simulink model "ssc_1C_Model_NT_MATLABfunc_est"  (R2019a)
settings: Solver=VariableStepAuto  StartTime=0  StopTime=150  FixedStep=0.05  RelTol=1e-4
undefined symbols (not defined in the file): C1_LUT, Capacity, Em_LUT, h, R0_LUT, R1_LUT, sigbuilder_block, SOC_LUT
libraries: nesl_utility x8, fl_lib x3
settings Model: OrderedModelArguments=off  Creator=ekonu001  LastModifiedBy=ekonu001
settings DataIOCC: ExternalInput=t

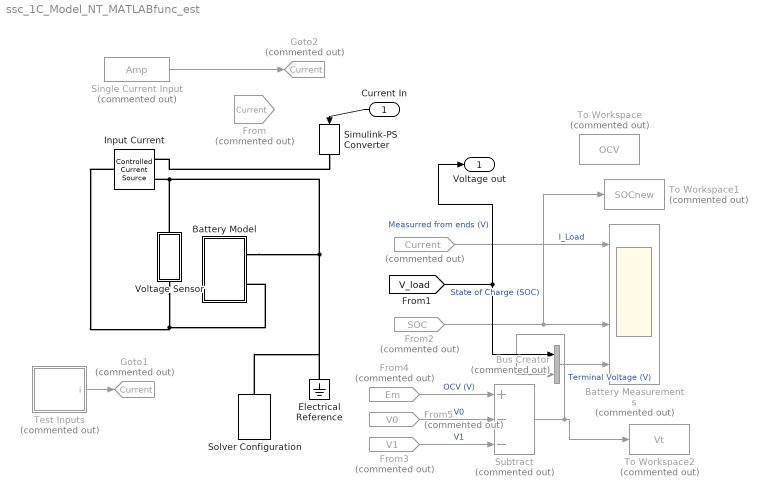
== system ssc_1C_Model_NT_MATLABfunc_est ==
  Current In : Inport
  " " : From  Commented=on  GotoTag=Current  TagVisibility=global
  Battery Measurements : Scope  Commented=on  NumInputPorts=4
  "Battery Model " : Subsystem
  Bus Creator : BusCreator  Commented=on  Inputs=2
  Electrical Reference : fl_lib/Electrical/Electrical Elements/Electrical Reference
  From : From  Commented=on  GotoTag=Current  TagVisibility=global
  From2 : From  Commented=on  GotoTag=SOC  TagVisibility=global
  From3 : From  Commented=on  GotoTag=V1  TagVisibility=global
  From4 : From  Commented=on  GotoTag=Em  TagVisibility=global
  From5 : From  Commented=on  GotoTag=V0  TagVisibility=global
  Goto1 : Goto  Commented=on  GotoTag=Current  TagVisibility=global
  Goto2 : Goto  Commented=on  GotoTag=Current  TagVisibility=global
  Input Current : fl_lib/Electrical/Electrical Sources/Controlled Current Source
  Simulink-PS Converter : nesl_utility/Simulink-PS Converter  PhysicalDomain=network_engine_domain  SubClassName=ps_input  LeftPortType=input  RightPortType=output  PseudoPeriodic=off  Frequencies=[]  NoiseDistribution=none  NoiseParameters=[]  Unit=A  AffineConversion=off  FilteringAndDerivatives=zero  SimscapeFilterOrder=1  InputFilterTimeConstant=.001  UdotUserProvided=0
  Single Current Input : FromWorkspace  Commented=on  VariableName=Amp  SampleTime=h
  Solver Configuration : nesl_utility/Solver Configuration  PhysicalDomain=network_engine_domain  SubClassName=solver  LeftPortType=input  RightPortType=generic  Tones=[]  Harmonics=[]  SimulateNoise=off  Profile=off  UseLocalSampling=off  EnableSwitchedLinearOptims=on  FrequencyDomain=off  UseCCode=off  RelTol=0.001  AbsTol=1e-06  MinStep=1e-09  ToWorkspace=off  RevertToSquareIcSolve=off  NumHomotopyIterations=100  PhasorMode=off  PhasorModeNumHarmonics=1  DoDC=off  ResidualTolerance=1e-09  UseLocalSolver=off  LocalSolverChoice=NE_BACKWARD_EULER_ADVANCER  LocalSolverSampleTime=0.001  DoFixedCost=off  MaxNonlinIter=3  MaxModeIter=2  LinearAlgebra=auto  EquationFormulation=NE_TIME_EF  DelaysMemoryBudget=1024  AutomaticFiltering=on  FilteringTimeConstant=0.001  PartitionStorageMethod=AS_NEEDED  PartitionMemoryBudget=1024  PartitionMethod=ROBUST
  Subtract : Sum  Commented=on  Inputs=+--
  Test Inputs : Subsystem  Commented=on
  To Workspace : ToWorkspace  Commented=on  VariableName=OCV  SampleTime=h
      settings: Decimation=6  Save2DSignal=2-D array (concatenate along first dimension)
  To Workspace1 : ToWorkspace  Commented=on  VariableName=SOCnew  SampleTime=h
      settings: Decimation=4  Save2DSignal=2-D array (concatenate along first dimension)
  To Workspace2 : ToWorkspace  Commented=on  VariableName=Vt  SampleTime=h
      settings: Decimation=6  Save2DSignal=2-D array (concatenate along first dimension)
  Voltage Sensor : Subsystem
      mask Display: disp('V_load')
  Voltage out : Outport
  wires:
  Test Inputs/1(i) -> Goto1/1
  " "/1 -> Battery Measurements/1  "I_Load"
  From2/1 -> To Workspace1/1, Battery Measurements/3  "State of Charge (SOC)"
  From3/1 -> Subtract/3  "V1"
  From4/1 -> Subtract/1  "OCV (V)"
  Subtract/1 -> Bus Creator/2, To Workspace2/1  "Terminal Voltage (V)"
  From5/1 -> Subtract/2  "V0"
  Single Current Input/1 -> Goto2/1
  Bus Creator/1 -> Battery Measurements/4
  [V_load] -> Bus Creator/1, Voltage out/1  "Measurred from ends (V)"
  Current In/1 -> Simulink-PS Converter/1
  connections:
  "Battery Model "/LConn1 -- Solver Configuration/RConn1 -- Electrical Reference/LConn1 -- Voltage Sensor/LConn1 -- Input Current/RConn2
  Input Current/LConn1 -- Voltage Sensor/RConn1 -- "Battery Model "/LConn2
  Simulink-PS Converter/RConn1 -- Input Current/RConn1

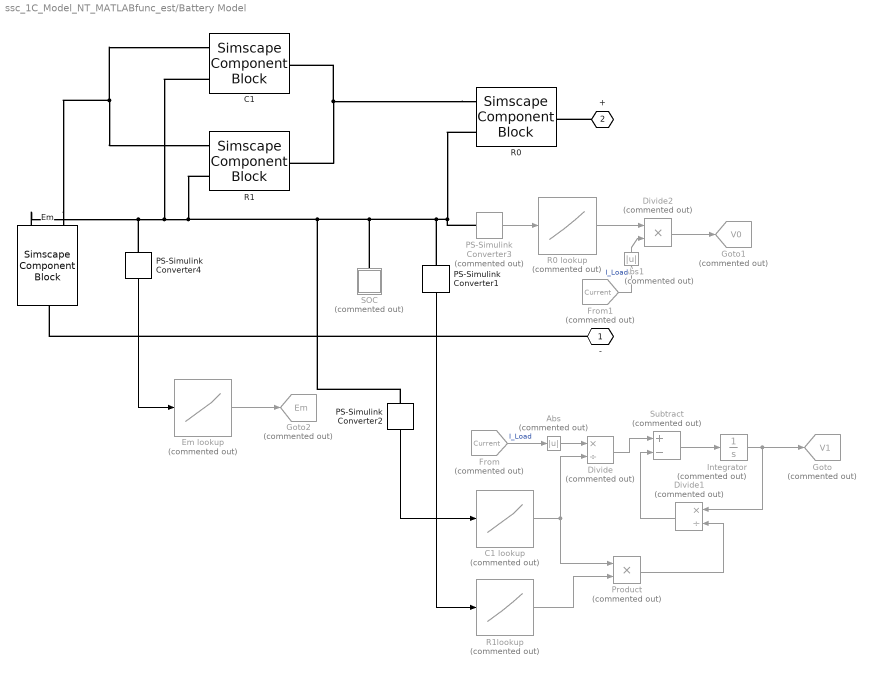
== system ssc_1C_Model_NT_MATLABfunc_est/Battery Model  ==
  " SOC " : Subsystem  Commented=on
  Abs : Abs  Commented=on
  Abs1 : Abs  Commented=on
  C1 : SimscapeComponentBlock  SourceFile=LiBatteryElements.C_table_1Temp  ComponentPath=LiBatteryElements.C_table_1Temp  ComponentVariants=LiBatteryElements.C_table_1Temp  ComponentVariantNames=C_table_1Temp  ClassName=C_table_1Temp  SchemaVersion=1  C_Table=C1_LUT F  SOC_Table=SOC_LUT  v0=0 V
      settings: CopyFcn=simscape.engine.sli.internal.componentblockcallback(gcbh,'COPY')  PreCopyFcn=simscape.engine.sli.internal.componentblockcallback(gcbh,'PRECOPY')  PreDeleteFcn=simscape.engine.sli.internal.componentblockcallback(gcbh,'PREDELETE')
      mask Type: C_table_1Temp
  C1 lookup : Lookup_n-D  Commented=on  NumberOfTableDimensions=1  BreakpointsForDimension1=SOC_LUT  BreakpointsForDimension2=[1:3]  Table=C1_LUT  InterpMethod=Linear Lagrange  InternalRulePriority=Speed  RndMeth=Simplest  InputSameDT=on
  Divide : Product  Commented=on  Inputs=*/
  Divide1 : Product  Commented=on  Inputs=*/
  Divide2 : Product  Commented=on  Inputs=**
  Em : SimscapeComponentBlock  SourceFile=LiBatteryElements.Em_table_1Temp  ComponentPath=LiBatteryElements.Em_table_1Temp  ComponentVariants=LiBatteryElements.Em_table_1Temp  ComponentVariantNames=Em_table_1Temp  ClassName=Em_table_1Temp  SchemaVersion=1  Em_Table=Em_LUT V  SOC_Table=SOC_LUT  C=Capacity hr*A  Qinit=Qe_init hr*A
      settings: CopyFcn=simscape.engine.sli.internal.componentblockcallback(gcbh,'COPY')  PreCopyFcn=simscape.engine.sli.internal.componentblockcallback(gcbh,'PRECOPY')  PreDeleteFcn=simscape.engine.sli.internal.componentblockcallback(gcbh,'PREDELETE')
      mask Type: Em_table_1Temp
  Em lookup : Lookup_n-D  Commented=on  NumberOfTableDimensions=1  BreakpointsForDimension1=SOC_LUT  BreakpointsForDimension2=[1:3]  Table=Em_LUT  InterpMethod=Linear Lagrange  InternalRulePriority=Speed  RndMeth=Simplest  InputSameDT=on
  From : From  Commented=on  GotoTag=Current
  From1 : From  Commented=on  GotoTag=Current
  Goto : Goto  Commented=on  GotoTag=V1  TagVisibility=global
  Goto1 : Goto  Commented=on  GotoTag=V0  TagVisibility=global
  Goto2 : Goto  Commented=on  GotoTag=Em  TagVisibility=global
  Integrator : Integrator  Commented=on
  PS-Simulink Converter1 : nesl_utility/PS-Simulink Converter  PhysicalDomain=network_engine_domain  SubClassName=ps_output  LeftPortType=input  RightPortType=output  PseudoPeriodic=off  Frequencies=[]  Unit=1  AffineConversion=off
  PS-Simulink Converter2 : nesl_utility/PS-Simulink Converter  PhysicalDomain=network_engine_domain  SubClassName=ps_output  LeftPortType=input  RightPortType=output  PseudoPeriodic=off  Frequencies=[]  Unit=1  AffineConversion=off
  PS-Simulink Converter3 : nesl_utility/PS-Simulink Converter  Commented=on  PhysicalDomain=network_engine_domain  SubClassName=ps_output  LeftPortType=input  RightPortType=output  PseudoPeriodic=off  Frequencies=[]  Unit=1  AffineConversion=off
  PS-Simulink Converter4 : nesl_utility/PS-Simulink Converter  PhysicalDomain=network_engine_domain  SubClassName=ps_output  LeftPortType=input  RightPortType=output  PseudoPeriodic=off  Frequencies=[]  Unit=1  AffineConversion=off
  Product : Product  Commented=on
  R0 : SimscapeComponentBlock  SourceFile=LiBatteryElements.R_table_1Temp  ComponentPath=LiBatteryElements.R_table_1Temp  ComponentVariants=LiBatteryElements.R_table_1Temp  ComponentVariantNames=R_table_1Temp  ClassName=R_table_1Temp  SchemaVersion=1  R_Table=R0_LUT Ohm  SOC_Table=SOC_LUT
      settings: CopyFcn=simscape.engine.sli.internal.componentblockcallback(gcbh,'COPY')  PreCopyFcn=simscape.engine.sli.internal.componentblockcallback(gcbh,'PRECOPY')  PreDeleteFcn=simscape.engine.sli.internal.componentblockcallback(gcbh,'PREDELETE')
      mask Type: R_table_1Temp
  R0 lookup : Lookup_n-D  Commented=on  NumberOfTableDimensions=1  BreakpointsForDimension1=SOC_LUT  BreakpointsForDimension2=[1:3]  Table=R0_LUT  InterpMethod=Linear Lagrange  InternalRulePriority=Speed  RndMeth=Simplest  InputSameDT=on
  "R1 " : SimscapeComponentBlock  SourceFile=LiBatteryElements.R_table_1Temp  ComponentPath=LiBatteryElements.R_table_1Temp  ComponentVariants=LiBatteryElements.R_table_1Temp  ComponentVariantNames=R_table_1Temp  ClassName=R_table_1Temp  SchemaVersion=1  R_Table=R1_LUT Ohm  SOC_Table=SOC_LUT
      settings: CopyFcn=simscape.engine.sli.internal.componentblockcallback(gcbh,'COPY')  PreCopyFcn=simscape.engine.sli.internal.componentblockcallback(gcbh,'PRECOPY')  PreDeleteFcn=simscape.engine.sli.internal.componentblockcallback(gcbh,'PREDELETE')
      mask Type: R_table_1Temp
  "R1lookup " : Lookup_n-D  Commented=on  NumberOfTableDimensions=1  BreakpointsForDimension1=SOC_LUT  BreakpointsForDimension2=[1:3]  Table=R1_LUT  InterpMethod=Linear Lagrange  InternalRulePriority=Speed  RndMeth=Simplest  InputSameDT=on
  Subtract : Sum  Commented=on  Inputs=+-
  - : PMIOPort  Tag=PMCPort  Side=Left
  + : PMIOPort  Tag=PMCPort  Port=2  Side=Left
  wires:
  PS-Simulink Converter1/1 -> "R1lookup "/1
  PS-Simulink Converter2/1 -> C1 lookup/1
  From/1 -> Abs/1  "I_Load"
  C1 lookup/1 -> Product/1, Divide/2
  "R1lookup "/1 -> Product/2
  Product/1 -> Divide1/2
  Divide/1 -> Subtract/1
  Divide1/1 -> Subtract/2
  Subtract/1 -> Integrator/1
  Integrator/1 -> Divide1/1, Goto/1
  PS-Simulink Converter3/1 -> R0 lookup/1
  From1/1 -> Abs1/1  "I_Load"
  R0 lookup/1 -> Divide2/1
  Divide2/1 -> Goto1/1
  Abs/1 -> Divide/1
  Abs1/1 -> Divide2/2
  PS-Simulink Converter4/1 -> Em lookup/1
  Em lookup/1 -> Goto2/1
  connections:
  Em/LConn1 -- C1/LConn1 -- "R1 "/LConn1
  +/RConn1 -- R0/RConn1
  R0/LConn1 -- "R1 "/RConn1 -- C1/RConn1
  -/RConn1 -- Em/RConn1
  Em/LConn2 -- PS-Simulink Converter4/LConn1 -- C1/LConn2 -- PS-Simulink Converter2/LConn1 -- R0/LConn2 -- PS-Simulink Converter3/LConn1 -- PS-Simulink Converter1/LConn1 -- " SOC "/LConn1 -- "R1 "/LConn2

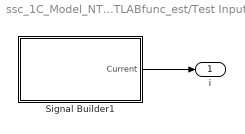
== system ssc_1C_Model_NT_MATLABfunc_est/Test Inputs ==
  Signal Builder1 : Subsystem  Tag=STV Subsys  LoadFcn=sigbuilder_block('load');  StartFcn=sigbuilder_block('start');  StopFcn=sigbuilder_block('stop');  ClipboardFcn=sigbuilder_block('clipboard');  mask(Sigbuilder block){tuvar=[0:10]}
      mask help: Simulink:masks:SigbuilderBlock_MD
      mask init:
      | if ~strcmp(get_param(bdroot(gcbh),'SimulationStatus'),'stopped') tuvar = sigbuilder_block('maskInit'); end
      settings: CopyFcn=sigbuilder_block('copy');  DeleteFcn=sigbuilder_block('delete');  ModelCloseFcn=sigbuilder_block('modelClose');  PreSaveFcn=sigbuilder_block('preSave');  PauseFcn=sigbuilder_block('pause');  ContinueFcn=sigbuilder_block('continue');  NameChangeFcn=sigbuilder_block('namechange');  OpenFcn=sigbuilder_block('open',[1877.25 80.25 755.25 277.5 ]);  CloseFcn=sigbuilder_block('close');
      mask Display: plot(0, 0, 100, 100,[2, 2, 32, 32, 2], [68, 8, 8, 68, 68],[32, 2], [38, 38], [32, 19, 2],[53, 60, 44], [32, 17, 17, 2],[16, 16, 31, 31]);txt = getActiveGroup(gcbh);text(2, 100, txt,'verticalAlignment', 'top');
  i : Outport
  wires:
  Signal Builder1/1(Current) -> i/1

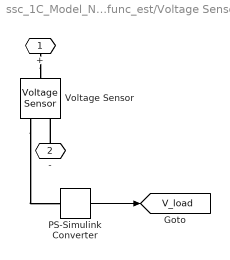
== system ssc_1C_Model_NT_MATLABfunc_est/Voltage Sensor ==
  PS-Simulink Converter : nesl_utility/PS-Simulink Converter  PhysicalDomain=network_engine_domain  SubClassName=ps_output  LeftPortType=input  RightPortType=output  PseudoPeriodic=off  Frequencies=[]  Unit=V  AffineConversion=off
  Voltage Sensor : fl_lib/Electrical/Electrical Sensors/Voltage Sensor
  + : PMIOPort  Side=Right
  - : PMIOPort  Port=2  Side=Left
  tag scope: V_load=global
  wires:
  PS-Simulink Converter/1 -> [V_load]
  connections:
  Voltage Sensor/RConn1 -- PS-Simulink Converter/LConn1
  +/RConn1 -- Voltage Sensor/LConn1
  -/RConn1 -- Voltage Sensor/RConn2

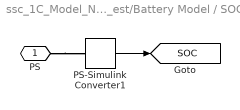
== system ssc_1C_Model_NT_MATLABfunc_est/Battery Model / SOC  ==
  PS-Simulink Converter1 : nesl_utility/PS-Simulink Converter  PhysicalDomain=network_engine_domain  SubClassName=ps_output  LeftPortType=input  RightPortType=output  PseudoPeriodic=off  Frequencies=[]  Unit=1  AffineConversion=off
  PS : PMIOPort  Side=Left
  tag scope: SOC=global
  wires:
  PS-Simulink Converter1/1 -> [SOC]
  connections:
  PS/RConn1 -- PS-Simulink Converter1/LConn1

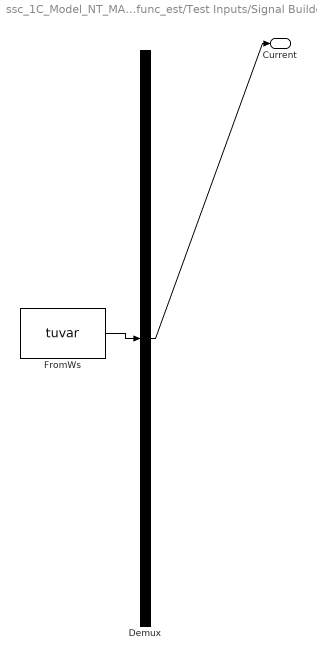
== system ssc_1C_Model_NT_MATLABfunc_est/Test Inputs/Signal Builder1 ==
  Demux : Demux  Tag=STV Demux  Outputs=1
  FromWs : FromWorkspace  Tag=STV FromWs  VariableName=tuvar  SampleTime=0
      SigBuilderData=|
      | common.afterFinalStr = 'Extrapolate'
      | common.sampleTime = '0'
      | dataSet.timeRange = [0 150]
      | dataSet.name = 'Sim Flight'
      | sbobj.Name = 'Signal Builder'
      | sbobj.Groups.Name = 'Sim Flight'
      | sbobj.Groups.Signals.Name = 'Current'
      | sbobj.Groups.Signals.XData = [0 2 5 49 49 150]
      | sbobj.Groups.Signals.YData = [-1.2 -12.3 -7.2 -8.2 -7.95 -8.15]
      | sbobj.Groups.TimeRange = [0 150]
  Current : Outport
  wires:
  FromWs/1 -> Demux/1
  Demux/1 -> Current/1
